simulink model "lab_2_3"  (R2016a)
settings: Solver=VariableStepAuto  StartTime=0.0  StopTime=10.0  RelTol=1e-3
settings Model: Creator=ms36124  LastModifiedBy=ms36124

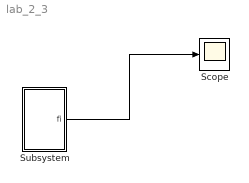
== system lab_2_3 ==
  Scope : Scope
  Subsystem : Subsystem  mask{m=10, k=1, l=3, g=10, fi0=90}
  wires:
  Subsystem/1("fi ") -> Scope/1

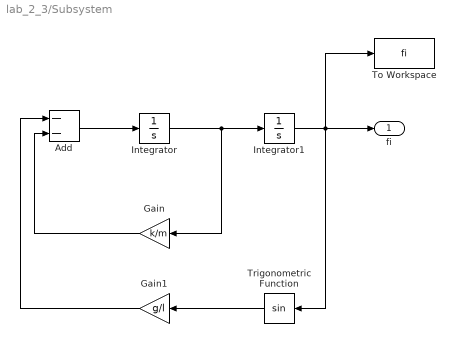
== system lab_2_3/Subsystem ==
  Add : Sum  Inputs=--
  Gain : Gain  Gain=k/m
  Gain1 : Gain  Gain=g/l
  Integrator : Integrator
  Integrator1 : Integrator  InitialCondition=fi0*pi/180
  To Workspace : ToWorkspace  VariableName=fi  SampleTime=-1
  Trigonometric Function : Trigonometry
  "fi " : Outport
  wires:
  Trigonometric Function/1 -> Gain1/1
  Integrator/1 -> Gain/1, Integrator1/1
  Add/1 -> Integrator/1
  Integrator1/1 -> To Workspace/1, "fi "/1, Trigonometric Function/1
  Gain1/1 -> Add/1
  Gain/1 -> Add/2
